simulink model "Final_Real_Model"  (R2023b)
settings: Solver=FixedStepAuto  StartTime=0.0  StopTime=2  FixedStep=0.01  RelTol=1e-3  EnableMultiTasking=on
libraries: arduinolib x3, arduinosensorlib x1, simulink x1
settings Model: NumberOfSteps=2  ExtModeTrigDuration=2  Creator=Taha  LastModifiedBy=Taha
settings OptimizationCC: EnhancedBackFolding=on  PassReuseOutputArgsAs=Individual arguments  ZeroExternalMemoryAtStartup=off  ZeroInternalMemoryAtStartup=off  MaxStackSize=64  OptimizeBlockOrder=speed  DifferentSizesBufferReuse=on  OptimizationCustomize=off  EfficientTunableParamExpr=on
settings DebuggingCC: ParameterPrecisionLossMsg=none  ParameterTunabilityLossMsg=error
settings HardwareCC: ProdBitPerInt=16  ProdBitPerPointer=16  ProdBitPerSizeT=16  ProdBitPerPtrDiffT=16  ProdLargestAtomicFloat=None  ProdWordSize=8  ProdHWDeviceType=Atmel->AVR  UseEmbeddedCoderFeatures=off  UseSimulinkCoderFeatures=off
settings SFSimCC: MATLABDynamicMemAlloc=off
settings RTWCC: Description=Embedded Coder  SystemTargetFile=ert.tlc  HardwareBoard=Arduino Uno  TemplateMakefile=ert_default_tmf  RTWVerbose=off  Toolchain=Arduino AVR  BuildConfiguration=Faster Runs
settings CodeAppCC: ForceParamTrailComments=on  OperatorAnnotations=on  SimulinkDataObjDesc=on  SFDataObjDesc=on  InsertBlockDesc=on
settings ERTTargetCC: SupportContinuousTime=on  SupportNonInlinedSFcns=on  SupportVariableSizeSignals=on  ExtModeTransport=3  ExtModeStaticAlloc=on  ExtModeAutomaticAllocSize=off  ExtModeStaticAllocSize=250  ExtModeMexFile=ext_xcp  ExtModeIntrfLevel=Level2 - Open  ERTSrcFileBannerTemplate=codertarget_code_template.cgt  ERTHdrFileBannerTemplate=codertarget_code_template.cgt  ERTDataSrcFileTemplate=codertarget_code_template.cgt  ERTDataHdrFileTemplate=codertarget_code_template.cgt

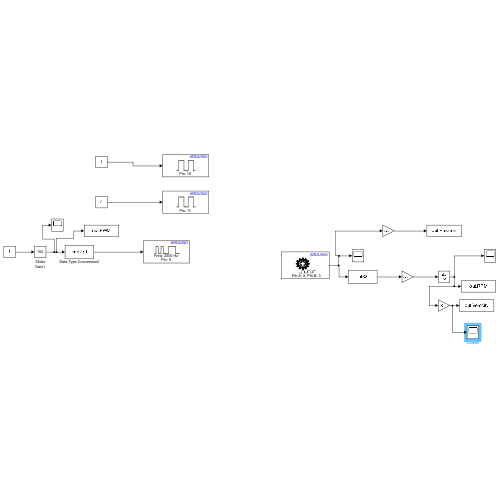
[thumbnail: Simulink's stored preview of the top-level diagram]
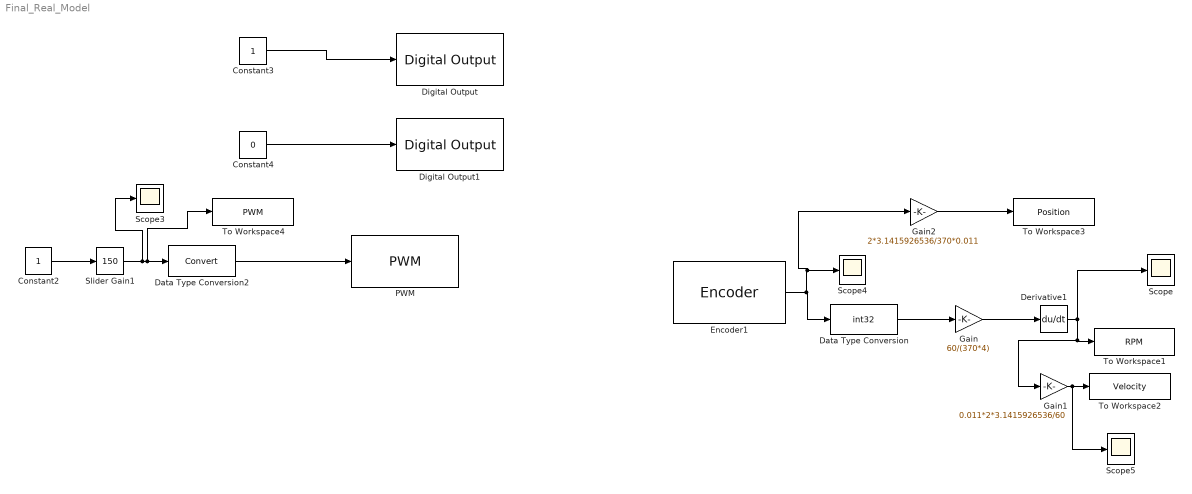
== system Final_Real_Model ==
  Constant2 : Constant
  Constant3 : Constant
  Constant4 : Constant  Value=0
  Data Type Conversion : DataTypeConversion  OutDataTypeStr=int32  SaturateOnIntegerOverflow=off  RndMeth=Floor
  Data Type Conversion2 : DataTypeConversion  SaturateOnIntegerOverflow=off  RndMeth=Floor
  Derivative1 : Derivative
  Digital Output : arduinolib/Digital Output  pinNumber=10  Direction=output  blockPlatform=arduino
  Digital Output1 : arduinolib/Digital Output  pinNumber=11  Direction=output  blockPlatform=arduino
  Encoder1 : arduinosensorlib/Encoder  InputA=2  InputB=3  Mode=No reset  SampleTime=-1
  Gain : Gain  Gain=60/(370*4)  OutDataTypeStr=double
  Gain1 : Gain  Gain=0.011*2*3.1415926536/60  ParamDataTypeStr=single  OutDataTypeStr=double
  Gain2 : Gain  Gain=2*3.1415926536/370*0.011  ParamDataTypeStr=single  OutDataTypeStr=double
  PWM : arduinolib/PWM  pinNumber=9  frequencyType=Specify  desiredFrequency=2000  achievableFrequency=2000
  Scope{,3..5} (4 alike) : Scope
  Slider Gain1 : simulink/Math Operations/Slider Gain  gain=150  low=0  high=255
  To Workspace1 : ToWorkspace  VariableName=RPM  SampleTime=-1
      settings: Save2DSignal=2-D array (concatenate along first dimension)
  To Workspace2 : ToWorkspace  VariableName=Velocity  SaveFormat=Timeseries  SampleTime=-1
      settings: Save2DSignal=2-D array (concatenate along first dimension)
  To Workspace3 : ToWorkspace  VariableName=Position  SaveFormat=Timeseries  SampleTime=-1
  To Workspace4 : ToWorkspace  VariableName=PWM  SampleTime=-1
      settings: Save2DSignal=2-D array (concatenate along first dimension)
  wires:
  Constant2/1 -> Slider Gain1/1
  Data Type Conversion2/1 -> PWM/1
  Slider Gain1/1 -> Scope3/1, To Workspace4/1, Data Type Conversion2/1
  Data Type Conversion/1 -> Gain/1
  Gain/1 -> Derivative1/1
  Derivative1/1 -> Gain1/1, To Workspace1/1, Scope/1
  Gain1/1 -> Scope5/1, To Workspace2/1
  Encoder1/1 -> Gain2/1, Scope4/1, Data Type Conversion/1
  Gain2/1 -> To Workspace3/1
  Constant4/1 -> Digital Output1/1
  Constant3/1 -> Digital Output/1
